simulink library "SvnInfo"  (R2022b)
settings: Solver=VariableStepAuto  StartTime=0.0  StopTime=10.0  RelTol=1e-3
undefined symbols (not defined in the file or in its folder): constDiagram, constRepo, constRev, constTag
libraries: StateVar x4, HandyTextFile x2, FeaturePath x1
settings Model: Creator=kl13806  LastModifiedBy=kl13806
settings DebuggingCC: UnconnectedInputMsg=warning  UnconnectedOutputMsg=warning  UnconnectedLineMsg=warning
settings ModelReferenceCC: EnableRefExpFcnMdlSchedulingChecks=on
settings RTWCC: DLArmComputeVersion=19.05

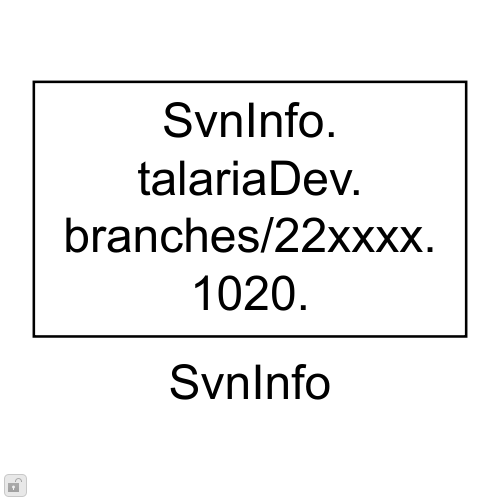
[thumbnail: Simulink's stored preview of the top-level diagram]
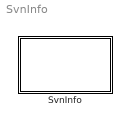
== system SvnInfo ==
  SvnInfo : Subsystem  mask{TriggerInit=[-230 41 -140 94], Config=[], FeatureName=Svn}
      mask prompts: Config "SvnInfoConfig"; FeatureName "Feature path name:"
      mask init:
      | blkh=gcbh;
      | Config=BTConfig.Assert(blkh,Config);
      | Config.Validate();
      | 
      | % Retrieve the Tsp Data
      | [constDiagram,constRepo,constTag,constRev] = ...
      |     SvnInfoMask.DoInit(blkh,Config);
      | 
      | % Create an icon display text string with no zeros
      | iconText = [constDiagram,newline,constRepo,newline,constTag,newline,constRev];
      | iconText(iconText==0)=[];
      | 
      | BTConfig.InitSetFeatureIfPresent(blkh,'FeatureName');
      settings: MoveFcn=SvnInfoMask.CB_TriggerInit(gcbh);
      mask Callback Config: BTConfig.CallbackHideIfPresent(gcbh,{'FeatureName'});
      mask TypeOptions FeatureName: FeaturePath/FeatureName
      mask Display: disp(iconText)

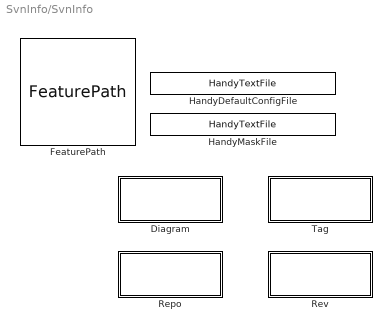
== system SvnInfo/SvnInfo ==
  Diagram : Subsystem  Variant=on
  FeaturePath : FeaturePath/FeaturePath  FeatureName=Svn  IsGroup=off  GroupNumber=-1  IsModule=off  TriggerInit=[170 -121 285 -14]
      settings: SourceProductName=Bose Talaria
  HandyDefaultConfigFile : HandyTextFile/HandyTextFile  TemplateSource=Config  FileSuffix=Init  OpenDialogOnLoad=off  UseThisBlockName=off  TheDefaultText=|  ShowInLibBrowser=on
      | % $(FILENAME) Setup model parameters for each "Init" callback (e.g. update diagram)
      | sample_rate_in_hertz = 44100;
      | frame_size = 32;
      | sysin_channel_count = 2;
      settings: SourceProductName=Bose Talaria
  HandyMaskFile : HandyTextFile/HandyTextFile  TemplateSource=Mask  FileSuffix=Init  OpenDialogOnLoad=off  UseThisBlockName=off  TheDefaultText=|  ShowInLibBrowser=on
      | % $(FILENAME) Setup model parameters for each "Init" callback (e.g. update diagram)
      | sample_rate_in_hertz = 44100;
      | frame_size = 32;
      | sysin_channel_count = 2;
      settings: SourceProductName=Bose Talaria
  Repo : Subsystem  Variant=on
  Rev : Subsystem  Variant=on
  Tag : Subsystem  Variant=on

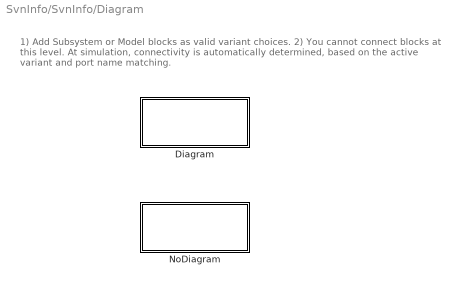
== system SvnInfo/SvnInfo/Diagram ==
  note: 1) Add Subsystem or Model blocks as valid variant choices.
      | 2) You cannot connect blocks at this level. At simulation, connectivity is automatically
      | determined, based on the active variant and port name matching.
  Diagram : Subsystem  VariantControl=(default)
  NoDiagram : Subsystem  VariantControl=Config.DiagramChars == 0

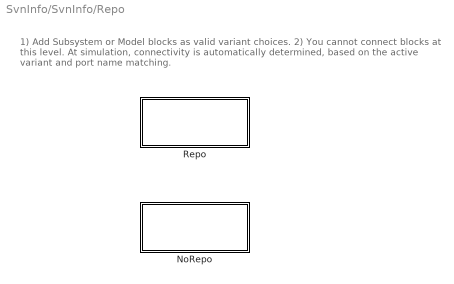
== system SvnInfo/SvnInfo/Repo ==
  note: 1) Add Subsystem or Model blocks as valid variant choices.
      | 2) You cannot connect blocks at this level. At simulation, connectivity is automatically
      | determined, based on the active variant and port name matching.
  NoRepo : Subsystem  VariantControl=Config.RepoChars == 0
  Repo : Subsystem  VariantControl=(default)

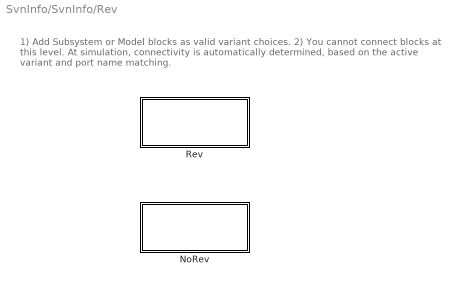
== system SvnInfo/SvnInfo/Rev ==
  note: 1) Add Subsystem or Model blocks as valid variant choices.
      | 2) You cannot connect blocks at this level. At simulation, connectivity is automatically
      | determined, based on the active variant and port name matching.
  NoRev : Subsystem  VariantControl=Config.RevChars == 0
  Rev : Subsystem  VariantControl=(default)

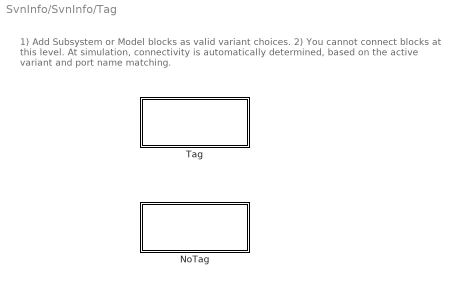
== system SvnInfo/SvnInfo/Tag ==
  note: 1) Add Subsystem or Model blocks as valid variant choices.
      | 2) You cannot connect blocks at this level. At simulation, connectivity is automatically
      | determined, based on the active variant and port name matching.
  NoTag : Subsystem  VariantControl=Config.TagChars == 0
  Tag : Subsystem  VariantControl=(default)

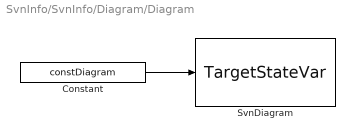
== system SvnInfo/SvnInfo/Diagram/Diagram ==
  Constant : Constant  Value=constDiagram
  SvnDiagram : StateVar/TargetStateVar  TriggerInit=[190 61 330 129]  TspName=Diagram  StateName=Diagram  UseSameName=on  IfdefMacro='CAPTURE_CONSTANT_TSPS'
      settings: SourceProductName=Bose Talaria
  wires:
  Constant/1 -> SvnDiagram/1

== system SvnInfo/SvnInfo/Diagram/NoDiagram ==

== system SvnInfo/SvnInfo/Repo/NoRepo ==

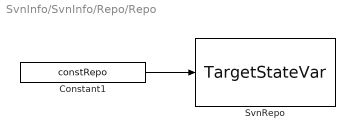
== system SvnInfo/SvnInfo/Repo/Repo ==
  Constant1 : Constant  Value=constRepo
  SvnRepo : StateVar/TargetStateVar  TriggerInit=[190 151 330 219]  TspName=Repo  StateName=Repo  UseSameName=on  IfdefMacro='CAPTURE_CONSTANT_TSPS'
      settings: SourceProductName=Bose Talaria
  wires:
  Constant1/1 -> SvnRepo/1

== system SvnInfo/SvnInfo/Rev/NoRev ==

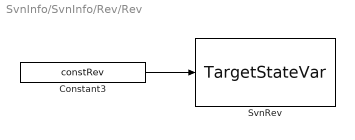
== system SvnInfo/SvnInfo/Rev/Rev ==
  Constant3 : Constant  Value=constRev
  SvnRev : StateVar/TargetStateVar  TriggerInit=[575 151 715 219]  TspName=Rev  StateName=Rev  UseSameName=on  IfdefMacro='CAPTURE_CONSTANT_TSPS'
      settings: SourceProductName=Bose Talaria
  wires:
  Constant3/1 -> SvnRev/1

== system SvnInfo/SvnInfo/Tag/NoTag ==

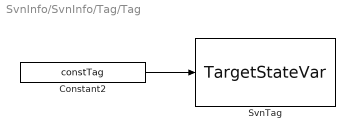
== system SvnInfo/SvnInfo/Tag/Tag ==
  Constant2 : Constant  Value=constTag
  SvnTag : StateVar/TargetStateVar  TriggerInit=[190 61 330 129]  TspName=Tag  StateName=Tag  UseSameName=on  IfdefMacro='CAPTURE_CONSTANT_TSPS'
      settings: SourceProductName=Bose Talaria
  wires:
  Constant2/1 -> SvnTag/1
